simulink model "model_2"  (R2023a)
settings: Solver=VariableStepAuto  StartTime=0.0  StopTime=50  RelTol=1e-3
values from neighbouring files (symbols this model uses):
  a = 1 / (p + q)    (= 0.111111111111)    [parameters.m]
  b = r + s    (= 3)    [parameters.m]
  c = p + q + r + s    (= 12)    [parameters.m]
libraries: simulink x1
settings Model: Creator=user  LastModifiedBy=user

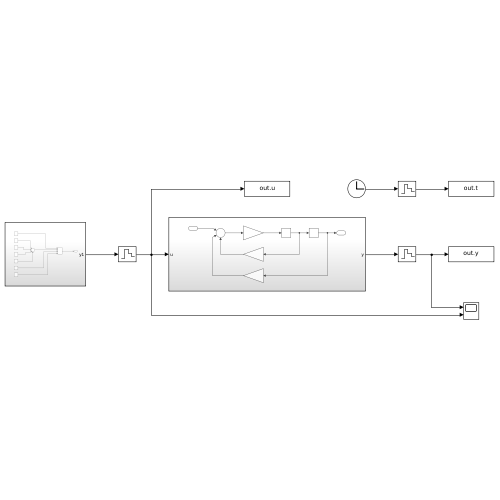
[thumbnail: Simulink's stored preview of the top-level diagram]
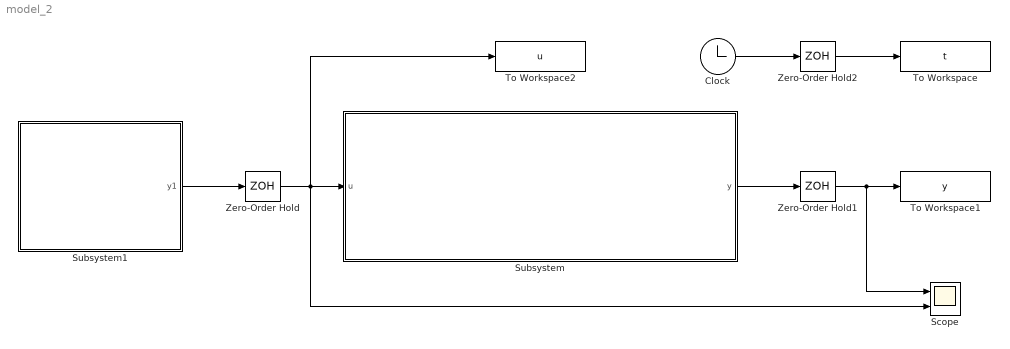
== system model_2 ==
  Clock : Clock
  Scope : Scope  NumInputPorts=2
  Subsystem : Subsystem
  Subsystem1 : Subsystem
  To Workspace : ToWorkspace  VariableName=t  SaveFormat=Timeseries  SampleTime=-1
  To Workspace1 : ToWorkspace  VariableName=y  SaveFormat=Timeseries  SampleTime=-1
  To Workspace2 : ToWorkspace  VariableName=u  SaveFormat=Timeseries  SampleTime=-1
  Zero-Order Hold : ZeroOrderHold  SampleTime=0.01
  Zero-Order Hold1 : ZeroOrderHold  SampleTime=0.01
  Zero-Order Hold2 : ZeroOrderHold  SampleTime=0.01
  wires:
  Zero-Order Hold/1 -> Subsystem/1(u), Scope/2, To Workspace2/1
  Subsystem/1(y) -> Zero-Order Hold1/1
  Subsystem1/1(y1) -> Zero-Order Hold/1
  Clock/1 -> Zero-Order Hold2/1
  Zero-Order Hold2/1 -> To Workspace/1
  Zero-Order Hold1/1 -> To Workspace1/1, Scope/1

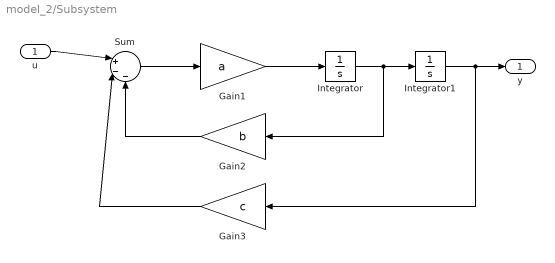
== system model_2/Subsystem ==
  u : Inport
  Gain1 : Gain  Gain=a
  Gain2 : Gain  Gain=b
  Gain3 : Gain  Gain=c
  Integrator : Integrator
  Integrator1 : Integrator
  Sum : Sum  Inputs=|+--
  y : Outport
  wires:
  Gain1/1 -> Integrator/1
  Gain2/1 -> Sum/3
  Sum/1 -> Gain1/1
  u/1 -> Sum/1
  Integrator/1 -> Integrator1/1, Gain2/1
  Integrator1/1 -> Gain3/1, y/1
  Gain3/1 -> Sum/2

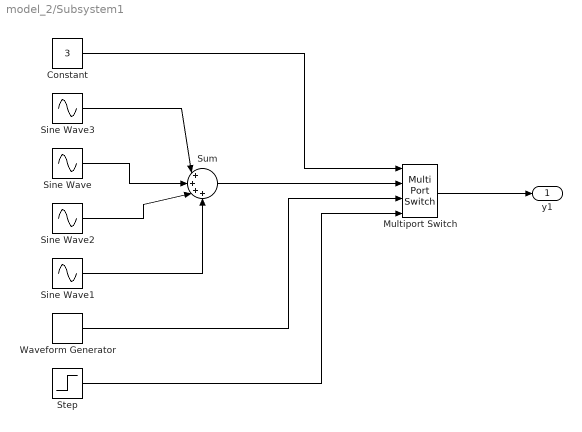
== system model_2/Subsystem1 ==
  Constant : Constant  Value=3
  Multiport Switch : MultiPortSwitch  SaturateOnIntegerOverflow=off  InputSameDT=off
  Sine Wave{,1..3} (4 alike) : Sin  SampleTime=0
  Step : Step  SampleTime=0
  Sum : Sum  Inputs=|++++
  Waveform Generator : simulink/Sources/Waveform Generator  OutMin=[]  OutMax=[]  OutDataTypeStr=double  SelectedSignal=1  BlockNames=MultiportSwitch_e3df3653d217406  SampleTime=0.1
  y1 : Outport
  wires:
  Sine Wave1/1 -> Sum/4
  Step/1 -> Multiport Switch/4
  Constant/1 -> Multiport Switch/1
  Multiport Switch/1 -> y1/1
  Sine Wave/1 -> Sum/2
  Sine Wave3/1 -> Sum/1
  Sum/1 -> Multiport Switch/2
  Sine Wave2/1 -> Sum/3
  Waveform Generator/1 -> Multiport Switch/3
